simulink model "14_Twelve_Pulse_Converter"  (R2014a)
settings: Solver=ode45  SolverMode=SingleTasking  StartTime=0.0  StopTime=0.08  RelTol=1e-3
undefined symbols (not defined in the file): D1, Delta, lagging
libraries: powerlib x22, powerlib_extras x1
settings Model: CovMetricSettings=dwe  CovHtmlReporting=off  covSaveCumulativeToWorkspaceVar=off  CovSaveSingleToWorkspaceVar=off  CovExternalEMLEnable=on  CovSFcnEnable=on  Creator=Vivek  LastModifiedBy=Vivek
settings DataIOCC: LimitDataPoints=off  SaveFormat=StructureWithTime
settings DebuggingCC: MergeDetectMultiDrivingBlocksExec=error  SolverPrmCheckMsg=none  FrameProcessingCompatibilityMsg=error  SFUnexpectedBacktrackingDiag=error  SFNoUnconditionalDefaultTransitionDiag=error
settings HardwareCC: ProdBitPerPointer=64  ProdLargestAtomicFloat=Float  ProdIntDivRoundTo=Zero  ProdEndianess=LittleEndian  ProdHWDeviceType=Specified
settings ModelReferenceCC: PropagateSignalLabelsOutOfModel=on
settings GRTTargetCC: TargetLangStandard=C99 (ISO)  GeneratePreprocessorConditionals=Use local settings
settings ConfigurationSet: Description=Simscape Multibody

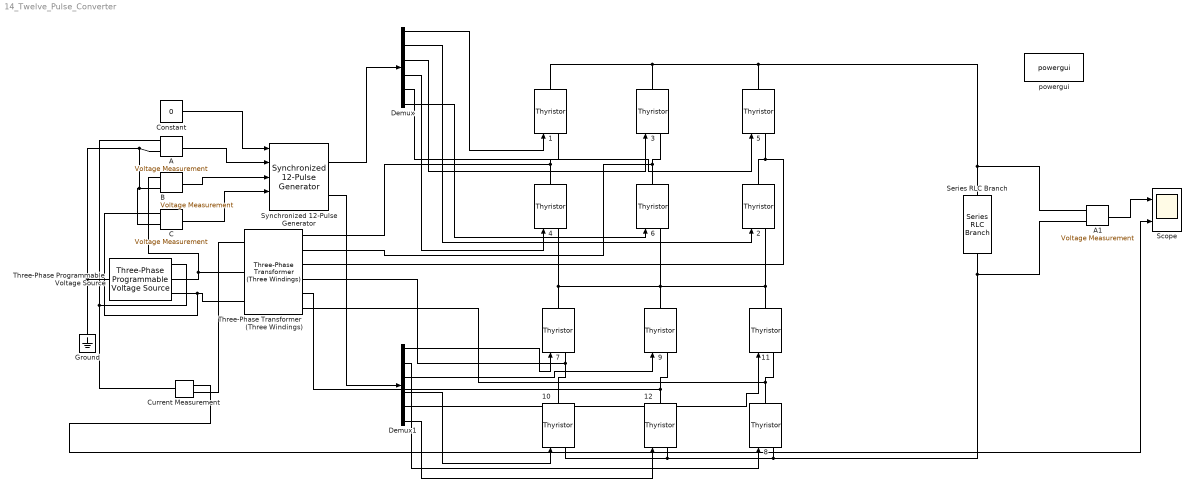
== system 14_Twelve_Pulse_Converter ==
  " Synchronized 12-Pulse Generator" : powerlib_extras/Control  Blocks/ Synchronized 12-Pulse Generator  Delta=D1 (lagging)  freq=50  pwidth=20  Double_Pulse=off
  {1..12} (12 alike) : powerlib/Power Electronics/Thyristor  Ron=0.001  Lon=0  Vf=0.8  IC=0  Rs=500  Cs=250e-9  Measurements=off
  A : powerlib/Measurements/Voltage Measurement  PhasorSimulation=off  OutputType=Complex  PSBequivalent=0
  A1 : powerlib/Measurements/Voltage Measurement  PhasorSimulation=off  OutputType=Complex  PSBequivalent=0
  B : powerlib/Measurements/Voltage Measurement  PhasorSimulation=off  OutputType=Complex  PSBequivalent=0
  C : powerlib/Measurements/Voltage Measurement  PhasorSimulation=off  OutputType=Complex  PSBequivalent=0
  Constant : Constant  Value=0
  Current Measurement : powerlib/Measurements/Current Measurement  PhasorSimulation=off  OutputType=Complex  PSBequivalent=0
  Demux : Demux  Outputs=6
  Demux1 : Demux  Outputs=6
  Ground : powerlib/Elements/Ground  LConnTagsString=a
  Scope : Scope  NumInputPorts=2
      settings: TimeRange=auto  MaxDataPoints=5000  SaveName=ScopeData  YMin=-2035.07058~-5  YMax=2038.09924~5  SampleTime=-1
  Series RLC Branch : powerlib/Elements/Series RLC Branch  LConnTagsString=__new0  RConnTagsString=__new0  BranchType=R  Resistance=10  Inductance=1e-3  SetiL0=off  InitialCurrent=0  Capacitance=1e-6  Setx0=off  InitialVoltage=0  Measurements=None
  Three-Phase Programmable Voltage Source : powerlib/Electrical Sources/Three-Phase Programmable Voltage Source  PositiveSequence="[440  0 50]"  VariationEntity=None  VariationType=Table of time-amplitude pairs  VariationTypeAlt=Step  VariationStep=0.5  VariationRate=10  VariationMagnitude=0.3  VariationFrequency=2  VariationTiming=[1 2]  VariationPhaseA=off  Amplitudes=[1 0.8 1.2 1.0]  TimeValues=[0 0.1 0.15 0.2]  HarmonicGeneration=off  HarmonicA=[3 0.2 -25 0]  HarmonicB=[2 0.15 35 2]  Timing="[0.05  3]"  BusType=swing  Pref=0  Qref=0  Qmin=-inf  Qmax=inf
  Three-Phase Transformer (Three Windings) : powerlib/Elements/Three-Phase Transformer (Three Windings)  Winding1Connection=Yg  Winding2Connection=Y  Winding3Connection=Delta (D1)  CoreType=Three single-phase transformers  SetSaturation=off  Hysteresis=off  DataFile='hysteresis'  SetInitialFlux=off  Measurements=None  UNITS=pu  NominalPower=[ 250e6 , 50]  Winding1=[ 400 , 0 , 0 ]  Winding2=[ 200 , 0 , 0 ]  Winding3=[ 200 , 0.001 , 0.00 ]  Rm=500  Lm=500  L0=0.5  Saturation=[ 0,0 ; 0.0024,1.2 ; 1.0,1.52 ]  InitialFluxes=[0.8 -0.8 0.7]  MoreParameters=off  BreakLoop=off  DataType=off  TransfoNumber=1
  powergui : powerlib/powergui  Priority=1  SimulationMode=Continuous  SampleTime=50e-6  frequency=60  Iterations=50  frequencyindice=50  Pbase=100e6  ErrMax=1e-4  UnitsV=kV  UnitsW=MW  buscounter=0  FunctionMessages=off  echomessages=off  EnableUseOfTLC=off  CurrentSourceSwitches=off  DisableSnubberDevices=off  DisableRonSwitches=off  DisableVfSwitches=off  DisplayEquations=off  SolverType=Tustin/Backward Euler (TBE)  Interpol=off  ExternalGateDelay=off  methode=off  Ts=100  x0status=blocks  SPID=on  SwTol=0  HookPort=off  RestoreLinks=warning  ResistiveCurrentMeasurement=off  Frange=[0:2:500]  Ylog=off  Xlog=on  ShowGrid=off  save=off  variable=ZData  structure=ScopeData  ZoomFFT=off  StartTime=0.04  cycles=1  DisplayStyle=1  fundamental=50  FreqAxis=on  MaxFrequency=1000  frequencyindicesteady=1  RmsSteady=1  display=off
  wires:
  A/1 -> " Synchronized 12-Pulse Generator"/2
  B/1 -> " Synchronized 12-Pulse Generator"/3
  C/1 -> " Synchronized 12-Pulse Generator"/4
  Constant/1 -> " Synchronized 12-Pulse Generator"/1
  " Synchronized 12-Pulse Generator"/1 -> Demux/1
  " Synchronized 12-Pulse Generator"/2 -> Demux1/1
  Demux/1 -> 1/1
  Demux/2 -> 2/1
  Demux/3 -> 3/1
  Demux/4 -> 4/1
  Demux/5 -> 5/1
  Demux/6 -> 6/1
  Demux1/1 -> 7/1
  Demux1/3 -> 9/1
  Demux1/5 -> 11/1
  Demux1/2 -> 8/1
  Demux1/4 -> 10/1
  Demux1/6 -> 12/1
  A1/1 -> Scope/1
  Current Measurement/1 -> Scope/2
  connections:
  1/LConn1 -- Three-Phase Transformer (Three Windings)/RConn1 -- 4/RConn1
  3/LConn1 -- Three-Phase Transformer (Three Windings)/RConn2 -- 6/RConn1
  5/LConn1 -- 2/RConn1 -- Three-Phase Transformer (Three Windings)/RConn3
  11/LConn1 -- Three-Phase Transformer (Three Windings)/RConn6 -- 8/RConn1
  9/LConn1 -- Three-Phase Transformer (Three Windings)/RConn5 -- 12/RConn1
  7/LConn1 -- 10/RConn1 -- Three-Phase Transformer (Three Windings)/RConn4
  9/RConn1 -- 7/RConn1 -- 4/LConn1 -- 6/LConn1 -- 2/LConn1 -- 11/RConn1
  Three-Phase Programmable Voltage Source/RConn2 -- B/LConn1 -- Three-Phase Transformer (Three Windings)/LConn2
  Three-Phase Programmable Voltage Source/RConn1 -- Current Measurement/LConn1 -- A/LConn1
  Three-Phase Programmable Voltage Source/RConn3 -- C/LConn1 -- Three-Phase Transformer (Three Windings)/LConn3
  Ground/LConn1 -- C/LConn2 -- B/LConn2 -- A/LConn2 -- Three-Phase Programmable Voltage Source/LConn1
  3/RConn1 -- 1/RConn1 -- A1/LConn1 -- Series RLC Branch/LConn1 -- 5/RConn1
  Series RLC Branch/RConn1 -- A1/LConn2 -- 10/LConn1 -- 12/LConn1 -- 8/LConn1
  Current Measurement/RConn1 -- Three-Phase Transformer (Three Windings)/LConn1
